simulink library "DipoleModel"  (R2020b)
settings: Solver=VariableStepAuto  StartTime=0.0  StopTime=10.0  RelTol=1e-3
values from neighbouring files (symbols this model uses):
  nmax = sqrt(numel(gh) + 1) - 1    [igrfsim.m]
undefined symbols (not defined in the file or in its folder): DipoleMod
settings Model: Creator=Dimitri  LastModifiedBy=colpari
settings SFSimCC: CustomCodeUndefinedFunction=UseInterfaceOnly

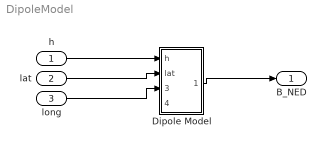
== system DipoleModel ==
  h : Inport
  "lat " : Inport  Port=2
  long : Inport  Port=3
  Dipole Model : Subsystem
  "B_NED " : Outport  VectorParamsAs1DForOutWhenUnconnected=off
  wires:
  h/1 -> Dipole Model/1(h)
  "lat "/1 -> Dipole Model/2("lat ")
  long/1 -> Dipole Model/3(long)
  Dipole Model/1("B_ECI ") -> "B_NED "/1

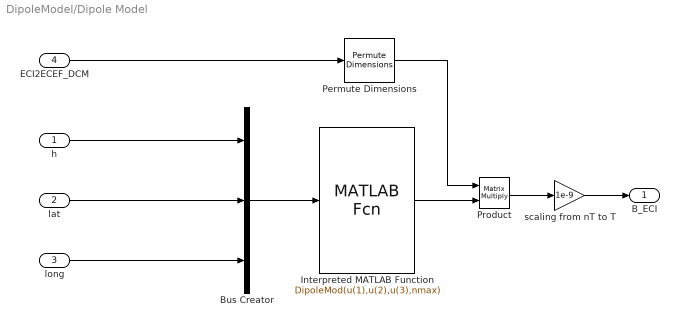
== system DipoleModel/Dipole Model ==
  h : Inport
  "lat " : Inport  Port=2
  long : Inport  Port=3
  ECI2ECEF_DCM : Inport  Port=4
  Bus Creator : BusCreator  Inputs=3
  Interpreted MATLAB Function : MATLABFcn  MATLABFcn=DipoleMod(u(1),u(2),u(3),nmax)
  Permute Dimensions : PermuteDimensions
  Product : Product  Multiplication=Matrix(*)
  scaling from nT to T : Gain  Gain=1e-9
  "B_ECI " : Outport  VectorParamsAs1DForOutWhenUnconnected=off
  wires:
  h/1 -> Bus Creator/1
  Interpreted MATLAB Function/1 -> Product/2
  scaling from nT to T/1 -> "B_ECI "/1
  long/1 -> Bus Creator/3
  "lat "/1 -> Bus Creator/2
  Bus Creator/1 -> Interpreted MATLAB Function/1
  ECI2ECEF_DCM/1 -> Permute Dimensions/1
  Permute Dimensions/1 -> Product/1
  Product/1 -> scaling from nT to T/1
